simulink model "q2_b"  (R2016a)
settings: Solver=VariableStepAuto  StartTime=0.0  StopTime=10.0  RelTol=1e-3
undefined symbols (not defined in the file): alpha, b, beta, k
settings Model: Creator=Huang Shemin  LastModifiedBy=Huang Shemin

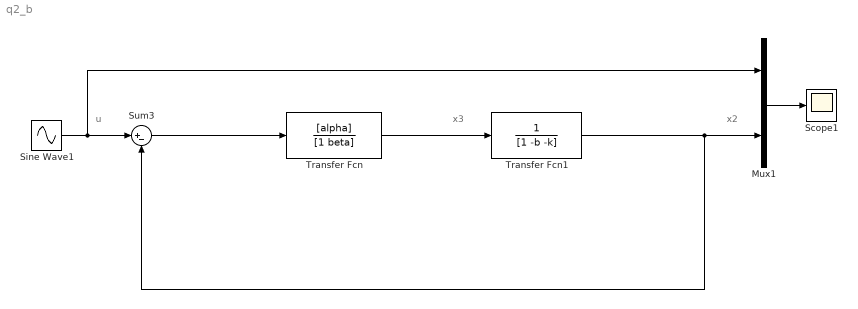
== system q2_b ==
  note: x2
  note: x3
  note: u
  Mux1 : Mux  Inputs=2
  Scope1 : Scope
  Sine Wave1 : Sin  Frequency=2*pi  SampleTime=0
  Sum3 : Sum  Inputs=|+-
  Transfer Fcn : TransferFcn  Numerator=[alpha]  Denominator=[1 beta]
  Transfer Fcn1 : TransferFcn  Denominator=[1 -b -k]
  wires:
  Transfer Fcn/1 -> Transfer Fcn1/1
  Sine Wave1/1 -> Mux1/1, Sum3/1
  Mux1/1 -> Scope1/1
  Transfer Fcn1/1 -> Mux1/2, Sum3/2
  Sum3/1 -> Transfer Fcn/1
